simulink model "simple_ASMC"  (R2022b)
settings: Solver=ode1  StartTime=0.0  StopTime=60  FixedStep=0.01  RelTol=1e-3
settings Model: Creator=Adan Daniel  LastModifiedBy=Adan Daniel

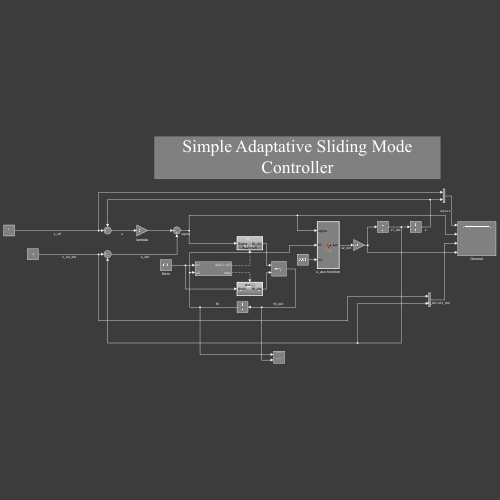
[thumbnail: Simulink's stored preview of the top-level diagram]
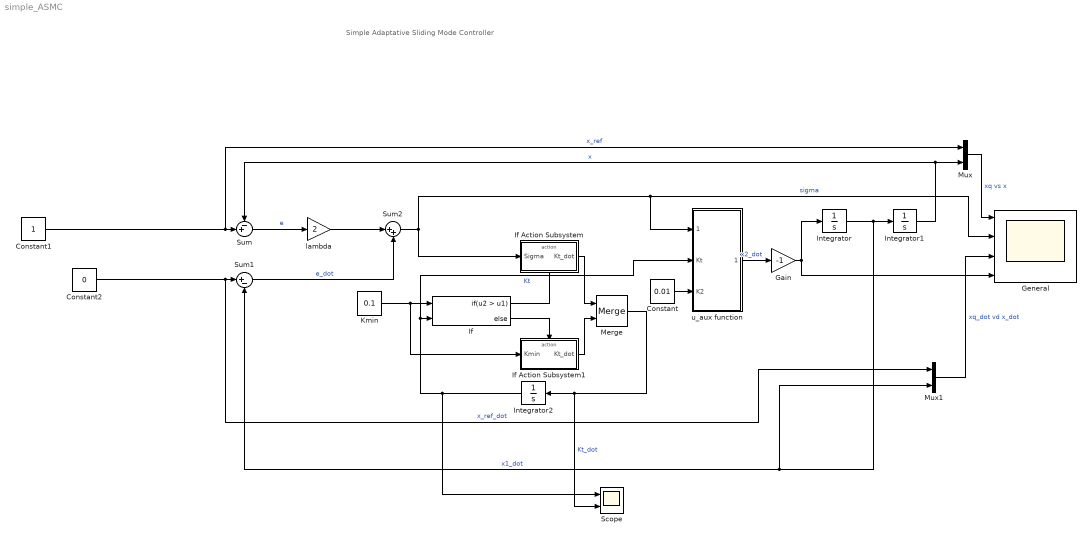
== system simple_ASMC ==
  note: Simple Adaptative Sliding Mode Controller
  Constant : Constant  Value=0.01
  Constant1 : Constant
  Constant2 : Constant  Value=0
  Gain : Gain  Gain=-1
  General : Scope  NumInputPorts=4
  If : If  NumInputs=2  IfExpression=u2 > u1
  If Action Subsystem : Subsystem  TreatAsAtomicUnit=on
  If Action Subsystem1 : Subsystem  TreatAsAtomicUnit=on
  Integrator : Integrator
  Integrator1 : Integrator
  Integrator2 : Integrator
  Kmin : Constant  Value=0.1
  Merge : Merge
  Mux : Mux  Inputs=2
  Mux1 : Mux  Inputs=2
  Scope : Scope  NumInputPorts=2
  Sum : Sum  Inputs=-+|
  Sum1 : Sum  Inputs=|+-
  Sum2 : Sum  Inputs=|++
  lambda : Gain  Gain=2
  u_aux function : MATLAB Function  TreatAsAtomicUnit=on
  wires:
  Mux1/1 -> General/3  "xq_dot vd x_dot"
  Constant2/1 -> Mux1/1, Sum1/1  "x_ref_dot"
  Integrator1/1 -> Mux/2, Sum/1  "x"
  Integrator/1 -> Sum1/2, Mux1/2, Integrator1/1  "x1_dot"
  Sum/1 -> lambda/1  "e"
  Sum1/1 -> Sum2/2  "e_dot"
  Sum2/1 -> If Action Subsystem/1(Sigma), u_aux function/1(sigma), General/2  "sigma"
  Mux/1 -> General/1  "xq vs x"
  lambda/1 -> Sum2/1
  u_aux function/1(u_aux) -> Gain/1  "x2_dot"
  Merge/1 -> Scope/2, Integrator2/1  "Kt_dot"
  Integrator2/1 -> Scope/1, u_aux function/2(Kt), If/2  "Kt"
  Kmin/1 -> If/1, If Action Subsystem1/1(Kmin)
  If/1 -> If Action Subsystem/Action
  If/2 -> If Action Subsystem1/Action
  If Action Subsystem/1(Kt_dot) -> Merge/1
  If Action Subsystem1/1(Kt_dot) -> Merge/2
  Constant/1 -> u_aux function/3(K2)
  Constant1/1 -> Mux/1, Sum/2  "x_ref"
  Gain/1 -> Integrator/1, General/4

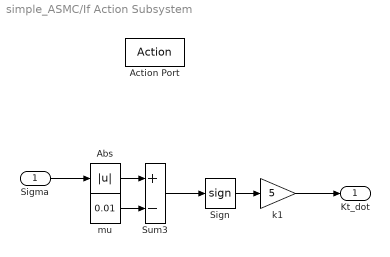
== system simple_ASMC/If Action Subsystem ==
  Sigma : Inport
  Action Port : ActionPort  ActionPortLabel=if(u2 > u1)
  Abs : Abs  SaturateOnIntegerOverflow=off
  Sign : Signum
  Sum3 : Sum  Inputs=+-
  k1 : Gain  Gain=5
  mu : Constant  Value=0.01
  Kt_dot : Outport
  wires:
  Sign/1 -> k1/1
  mu/1 -> Sum3/2
  Sum3/1 -> Sign/1
  Abs/1 -> Sum3/1
  k1/1 -> Kt_dot/1
  Sigma/1 -> Abs/1

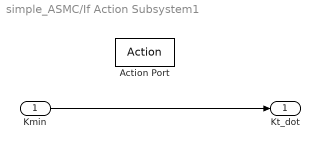
== system simple_ASMC/If Action Subsystem1 ==
  Kmin : Inport
  Action Port : ActionPort  ActionPortLabel=else
  Kt_dot : Outport
  wires:
  Kmin/1 -> Kt_dot/1

== matlab function simple_ASMC/u_aux function ==
  data: sigma input; u_aux output; Kt input; K2 input
function u_aux = fcn(sigma, Kt, K2)

u_aux = - Kt * (abs(sigma) ^ (0.5)) * sign(sigma) - K2 * sigma;
